simulink model "Test_Counter_3bit"  (R2016a)
settings: Solver=VariableStepAuto  StartTime=0.0  StopTime=100.0  RelTol=1e-3
libraries: commutil2 x1, simulink_extras x1, Clock_Lib x1
settings Model: Creator=Jozko Mrkvicka  LastModifiedBy=Jozko Mrkvicka

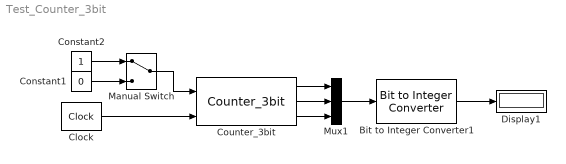
== system Test_Counter_3bit ==
  Bit to Integer Converter1 : commutil2/Bit to Integer Converter  nbits=3  bitOrder=MSB first  signedOutputValues=Unsigned  outDtype=uint8  outDtypeSigned=Inherit via internal rule
  Clock : simulink_extras/Flip Flops/Clock  period=2
  Constant1 : Constant  Value=0
  Constant2 : Constant
  Counter_3bit : Clock_Lib/Counter_3bit
  Display1 : Display
  Manual Switch : ManualSwitch
  Mux1 : Mux  Inputs=3
  wires:
  Clock/1 -> Counter_3bit/2
  Counter_3bit/1 -> Mux1/1
  Counter_3bit/3 -> Mux1/3
  Mux1/1 -> Bit to Integer Converter1/1
  Bit to Integer Converter1/1 -> Display1/1
  Manual Switch/1 -> Counter_3bit/1
  Counter_3bit/2 -> Mux1/2
  Constant2/1 -> Manual Switch/1
  Constant1/1 -> Manual Switch/2
